simulink model "Take_off_from_water"  (R2021b)
settings: Solver=FixedStepAuto  StartTime=0.0  StopTime=25  FixedStep=0.0001  RelTol=1e-3
settings Model: Creator=manavbathija  LastModifiedBy=manavbathija

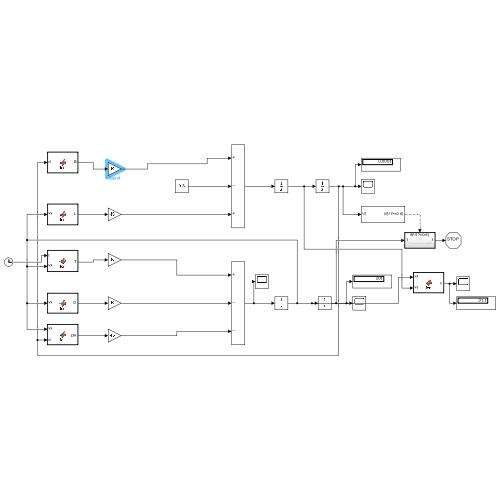
[thumbnail: Simulink's stored preview of the top-level diagram]
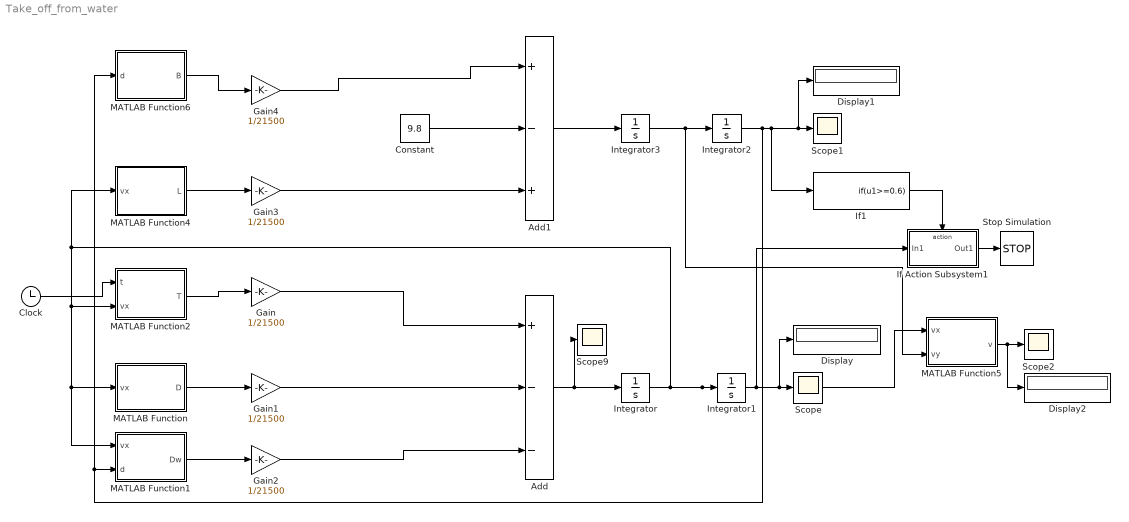
== system Take_off_from_water ==
  Add : Sum  Inputs=+--
  Add1 : Sum  Inputs=+-+
  Clock : Clock
  Constant : Constant  Value=9.8
  Display : Display
  Display1 : Display
  Display2 : Display
  Gain{,1..4} (5 alike) : Gain  Gain=1/21500
  If Action Subsystem1 : Subsystem  TreatAsAtomicUnit=on
  If1 : If  IfExpression=u1>=0.6  ShowElse=off
  Integrator : Integrator  InitialCondition=0.01
  Integrator1 : Integrator
  Integrator2 : Integrator
  Integrator3 : Integrator
  MATLAB Function : MATLAB Function  TreatAsAtomicUnit=on
  MATLAB Function1 : MATLAB Function  TreatAsAtomicUnit=on
  MATLAB Function2 : MATLAB Function  TreatAsAtomicUnit=on
  MATLAB Function4 : MATLAB Function  TreatAsAtomicUnit=on
  MATLAB Function5 : MATLAB Function  TreatAsAtomicUnit=on
  MATLAB Function6 : MATLAB Function  TreatAsAtomicUnit=on
  Scope{,1..2,9} (4 alike) : Scope
  Stop Simulation : Stop
  wires:
  If Action Subsystem1/1(Out1) -> Stop Simulation/1
  If1/1 -> If Action Subsystem1/Action
  MATLAB Function4/1(L) -> Gain3/1
  MATLAB Function2/1(T) -> Gain/1
  MATLAB Function/1(D) -> Gain1/1
  MATLAB Function1/1(Dw) -> Gain2/1
  Gain2/1 -> Add/3
  Add1/1 -> Integrator3/1
  Integrator3/1 -> MATLAB Function5/2(vy), Integrator2/1
  Add/1 -> Scope9/1, Integrator/1
  Integrator/1 -> MATLAB Function4/1(vx), MATLAB Function1/1(vx), MATLAB Function/1(vx), MATLAB Function2/2(vx), MATLAB Function5/1(vx), Integrator1/1
  Integrator1/1 -> If Action Subsystem1/1(In1), Display/1, Scope/1
  Integrator2/1 -> MATLAB Function6/1(d), MATLAB Function1/2(d), If1/1, Display1/1, Scope1/1
  MATLAB Function5/1(v) -> Display2/1, Scope2/1
  Clock/1 -> MATLAB Function2/1(t)
  MATLAB Function6/1(B) -> Gain4/1
  Gain4/1 -> Add1/1
  Gain/1 -> Add/1
  Constant/1 -> Add1/2
  Gain3/1 -> Add1/3
  Gain1/1 -> Add/2

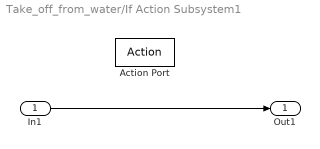
== system Take_off_from_water/If Action Subsystem1 ==
  In1 : Inport
  Action Port : ActionPort  ActionPortLabel=if(u1>=0.6)
  Out1 : Outport
  wires:
  In1/1 -> Out1/1

== matlab function Take_off_from_water/MATLAB Function ==
  data: vx input; D output
function D = fcn(vx)

D = 0.5*1.225*vx^2*156*(0.04+(1/(pi*8.5*0.7))*2.6^2);

== matlab function Take_off_from_water/MATLAB Function2 ==
  data: t input; vx input; T output
function T = fcn(t,vx)
rpm=1212*t/15;
P=14913*rpm*0.10472;
T= 2*0.8*P/vx;

== matlab function Take_off_from_water/MATLAB Function4 ==
  data: vx input; L output
function L = fcn(vx)
    L=0.5*1.225*vx^2*2.6*156;
end

== matlab function Take_off_from_water/MATLAB Function5 ==
  data: vx input; v output; vy input
function v = fcn(vx,vy)
v=sqrt(vx^2+vy^2);
end

== matlab function Take_off_from_water/MATLAB Function6 ==
  data: d input; B output
function B = fcn(d)
Swet=34.82345*exp(-19*d);
B=1029*9.8*Swet*(0.6-d);
end

== matlab function Take_off_from_water/MATLAB Function1 ==
  data: vx input; Dw output; d input
function Dw= fcn(vx,d)
Swet=34.82345*exp(-19*d);
Dw=0.03*Swet*vx^2;
end
